simulink model "PD"  (R2018b)
settings: Solver=VariableStepAuto  StartTime=0.0  StopTime=10  RelTol=1e-3
undefined symbols (not defined in the file): Kd, Kp, parameter_estimated, parameter_true
libraries: simulink x1
settings Model: Creator=giga4  LastModifiedBy=AmatoPi
settings DebuggingCC: UnderSpecifiedDimensionMsg=warning

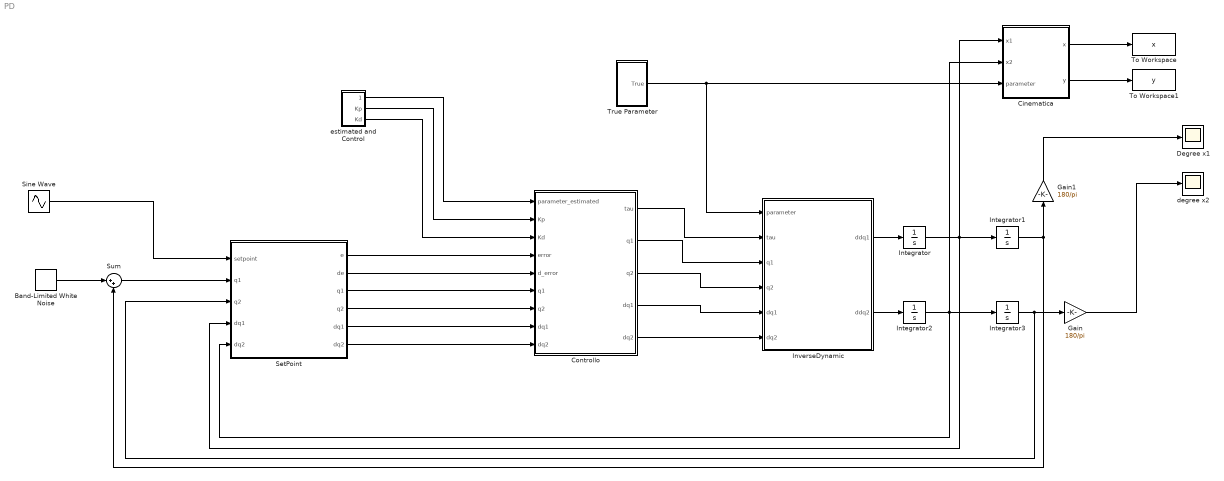
== system PD ==
  Band-Limited White Noise : simulink/Sources/Band-Limited White Noise  Cov=[0.01]  Ts=0.1  seed=[23341]
  Cinematica : MATLAB Function  TreatAsAtomicUnit=on
  Controllo : MATLAB Function  TreatAsAtomicUnit=on
  Degree x1 : Scope
  Gain : Gain  Gain=180/pi
  Gain1 : Gain  Gain=180/pi
  Integrator{,1..3} (4 alike) : Integrator
  InverseDynamic : MATLAB Function  TreatAsAtomicUnit=on
  SetPoint : MATLAB Function  TreatAsAtomicUnit=on
  Sine Wave : Sin  Amplitude=0.01  Frequency=100  SampleTime=0
  Sum : Sum  Inputs=|++
  To Workspace : ToWorkspace  VariableName=x  SaveFormat=Timeseries  SampleTime=-1
  To Workspace1 : ToWorkspace  VariableName=y  SaveFormat=Timeseries  SampleTime=-1
  True Parameter : Subsystem
  degree x2 : Scope
  estimated and Control : Subsystem
  wires:
  True Parameter/1(True) -> InverseDynamic/1(parameter), Cinematica/3(parameter)
  estimated and Control/1(Paramter Estimated) -> Controllo/1(parameter_estimated)
  estimated and Control/2(Kp) -> Controllo/2(Kp)
  estimated and Control/3(Kd) -> Controllo/3(Kd)
  Controllo/2(q1) -> InverseDynamic/3(q1)
  Controllo/3(q2) -> InverseDynamic/4(q2)
  Controllo/1(tau) -> InverseDynamic/2(tau)
  SetPoint/1(e) -> Controllo/4(error)
  SetPoint/2(de) -> Controllo/5(d_error)
  SetPoint/3(q1) -> Controllo/6("q1 ")
  SetPoint/4(q2) -> Controllo/7("q2 ")
  SetPoint/5(dq1) -> Controllo/8("dq1 ")
  SetPoint/6(dq2) -> Controllo/9("dq2 ")
  Controllo/4(dq1) -> InverseDynamic/5(dq1)
  Controllo/5(dq2) -> InverseDynamic/6(dq2)
  Sum/1 -> SetPoint/2("q1 ")
  InverseDynamic/1(ddq1) -> Integrator/1
  InverseDynamic/2(ddq2) -> Integrator2/1
  Integrator2/1 -> Cinematica/2(x2), SetPoint/5("dq2 "), Integrator3/1
  Gain1/1 -> Degree x1/1
  Sine Wave/1 -> SetPoint/1(setpoint)
  Integrator3/1 -> Gain/1, SetPoint/3("q2 ")
  Gain/1 -> degree x2/1
  Integrator/1 -> Cinematica/1(x1), Integrator1/1, SetPoint/4("dq1 ")
  Integrator1/1 -> Sum/2, Gain1/1
  Band-Limited White Noise/1 -> Sum/1
  Cinematica/1(x) -> To Workspace/1
  Cinematica/2(y) -> To Workspace1/1

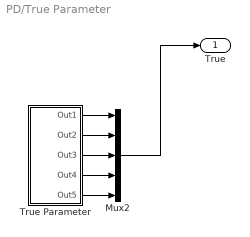
== system PD/True Parameter ==
  Mux2 : Mux  Inputs=5
  True Parameter : Subsystem
  True : Outport
  wires:
  True Parameter/3(Out3) -> Mux2/3
  True Parameter/4(Out4) -> Mux2/4
  True Parameter/5(Out5) -> Mux2/5
  Mux2/1 -> True/1
  True Parameter/1(Out1) -> Mux2/1
  True Parameter/2(Out2) -> Mux2/2

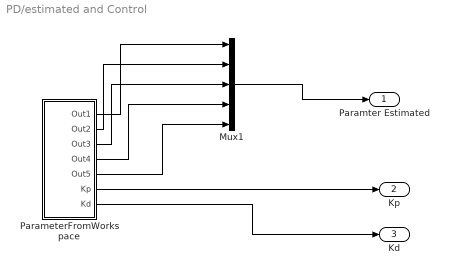
== system PD/estimated and Control ==
  Mux1 : Mux  Inputs=5
  "ParameterFromWorkspace " : Subsystem
  Paramter Estimated : Outport
  Kp : Outport  Port=2
  Kd : Outport  Port=3
  wires:
  "ParameterFromWorkspace "/1(Out1) -> Mux1/1
  "ParameterFromWorkspace "/4(Out4) -> Mux1/4
  "ParameterFromWorkspace "/7(Kd) -> Kd/1
  "ParameterFromWorkspace "/6("Kp ") -> Kp/1
  "ParameterFromWorkspace "/5(Out5) -> Mux1/5
  "ParameterFromWorkspace "/3(Out3) -> Mux1/3
  "ParameterFromWorkspace "/2(Out2) -> Mux1/2
  Mux1/1 -> Paramter Estimated/1

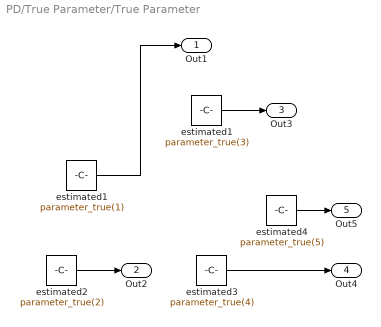
== system PD/True Parameter/True Parameter ==
  estimated1 : Constant  Value=parameter_true(3)
  "estimated1 " : Constant  Value=parameter_true(1)
  estimated2 : Constant  Value=parameter_true(2)
  estimated3 : Constant  Value=parameter_true(4)
  estimated4 : Constant  Value=parameter_true(5)
  Out1 : Outport
  Out2 : Outport  Port=2
  Out3 : Outport  Port=3
  Out4 : Outport  Port=4
  Out5 : Outport  Port=5
  wires:
  "estimated1 "/1 -> Out1/1
  estimated2/1 -> Out2/1
  estimated1/1 -> Out3/1
  estimated4/1 -> Out5/1
  estimated3/1 -> Out4/1

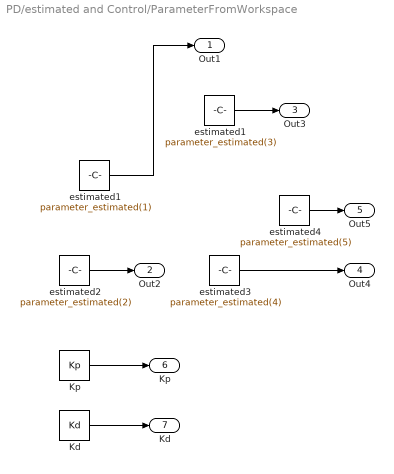
== system PD/estimated and Control/ParameterFromWorkspace  ==
  "Kd " : Constant  Value=Kd
  Kp : Constant  Value=Kp
  estimated1 : Constant  Value=parameter_estimated(3)
  "estimated1 " : Constant  Value=parameter_estimated(1)
  estimated2 : Constant  Value=parameter_estimated(2)
  estimated3 : Constant  Value=parameter_estimated(4)
  estimated4 : Constant  Value=parameter_estimated(5)
  Out1 : Outport
  Out2 : Outport  Port=2
  Out3 : Outport  Port=3
  Out4 : Outport  Port=4
  Out5 : Outport  Port=5
  "Kp " : Outport  Port=6
  Kd : Outport  Port=7
  wires:
  "estimated1 "/1 -> Out1/1
  estimated2/1 -> Out2/1
  estimated1/1 -> Out3/1
  estimated4/1 -> Out5/1
  estimated3/1 -> Out4/1
  Kp/1 -> "Kp "/1
  "Kd "/1 -> Kd/1

== matlab function PD/InverseDynamic ==
  data: parameter input; tau input; ddq1 output; q1 input; q2 input; dq1 input; dq2 input; ddq2 output
function [ddq1,ddq2] = Inv_Dynamic(parameter,tau,q1,q2,dq1,dq2)

    [B,C,G] = Generatore_Dinamica_SIMULINK(parameter,q1,q2,dq1,dq2);
    
    dq = [dq1,dq2]';
    ddq = B\(tau-C*dq-G); %inv(B)*(tau-C*dq-G);
    
    ddq1 = ddq(1);
    ddq2 = ddq(2);
    
end

== matlab function PD/Controllo ==
  data: parameter_estimated input; Kp input; Kd input; error input; d_error input; tau output; q1 input; q2 input; q1 output; q2 output; dq1 input; dq2 input; dq1 output; dq2 output
function [tau,q1,q2,dq1,dq2] = PID(parameter_estimated,Kp,Kd,error,d_error,q1,q2,dq1,dq2)


    [B,C,G] = Generatore_Dinamica_SIMULINK(parameter_estimated,q1,q2,dq1,dq2);
   
    
    tau = [0; Kp*error+Kd*d_error]+G;

end

== matlab function PD/SetPoint ==
  data: setpoint input; q1 input; e output; q2 input; de output; q1 output; q2 output; dq1 input; dq2 input; dq1 output; dq2 output
function [e,de,q1,q2,dq1,dq2] = generatore_Errore(setpoint,q1,q2,dq1,dq2)
    %Il controllo del PD si basa sull'angolo q1
    
    e =  setpoint-q1;
    de = setpoint-dq1;
    
end

== matlab function PD/Cinematica ==
  data: x1 input; x output; x2 input; parameter input; y output
function [x,y] = fcn(x1,x2,parameter)
    
    L = parameter(1);

    T = [ cos(x1 + x2), -sin(x1 + x2), 0, -L*sin(x1);
          sin(x1 + x2),  cos(x1 + x2), 0,  L*cos(x1);
                   0,             0, 1,          0;
                   0,             0, 0,          1];
               
    x = T(1,4);
    y = T(2,4);   
  
  
end
